simulink model "PCT_model_OG_2"  (R2021a)
settings: Solver=VariableStepAuto  StartTime=0.0  StopTime=10.0  RelTol=1e-3
undefined symbols (not defined in the file or in its folder): Disk, Floor, to, wo, X, Y, Z
libraries: sm_lib x66, nesl_utility x16, Contact_Forces_Lib x1, simulink x1, Parts_Lib x1, Multibody_Multiphysics_Lib x1, pid_lib x1
(part 3 of 3)

== matlab function PCT_model_OG_2/MATLAB Function2 ==
  data: cv input; dt input; cv output; g input; angley1 input; y1 input; y2 input
function cv = fcn(cv,dt,g,angley1,y1,y2)

            a_mult_t=dt*g*cos(angley1);
        %
            if y1>y2
            cv = cv+a_mult_t*sin(angley1);
        else %y2>y1
            cv = cv+a_mult_t*cos(angley1-pi/2);
        end
            %}
         %cv = cv+a_mult_t*sin(angley1);
end

== matlab function PCT_model_OG_2/MATLAB Function3 ==
  data: y1 input; angley1 output; y2 input; angley2 output; angley3 output; x1 input; x2 input
    function [angley1,angley2,angley3] = find_angleys(y1,y2,x1,x2)


    if y1>y2
        %use value set 1
        angley1=x1(1)+pi/2;  %mtrig manipulation to put in right quadrant
        angley2=0.5*pi-angley1; %internal angles of a right-angle-triangle
        angley3=x1(2);
    else %y2>=y1
        %use value set 2
        angley1=pi/2-x2(1);  %mtrig manipulation to put in right quadrant???
        angley2= -(0.5*pi-(pi-angley1)); %internal angles of a right-angle-triangle
        angley3=x2(2);
    end
        
end

== matlab function PCT_model_OG_2/MATLAB Function4 ==
  data: u1 input; y output; y1 input; a input; a output
function [y,a] = choose_u1(u1,y1,a)

if a==0
    y=u1;
    a=1;
else
    y=u1+y1;
end

end

== matlab function PCT_model_OG_2/MATLAB Function5 ==
  data: u2 input; y output; y2 input; b input
function y = choose_u2(u2,y2,b)

if b==0
    y=u2;
    b=1;
else
    y=u2+y2;
end

end
